simulink model "qpskUpdate"  (Simulink 9.2)
settings: Solver=FixedStepDiscrete  StartTime=0.0  StopTime=inf  RelTol=1e-3  AbsTol=1e-6
PreLoadFcn:
  | EbNo=3;maxNumErrs=100;maxNumBits=1e8;M=8;Tsym=.2;
model workspace: external: MATLAB Code (data not in the file)
libraries: commutil2 x2, commsink2 x2, commdigbbndpm3 x2, commchan3 x1, commrandsrc3 x1
Description:
  | Gray Coded 8-PSK
  | 
  | This model shows a communications link using Gray-coded 8-PSK modulation.
CloseFcn:
  | clear graySER grayBER graySigsOut EbNo maxNumErrs maxNumBits M Tsym
settings Model: RequirementInfo=9  Creator=The MathWorks, Inc.  LastModifiedBy=Milind  ExtModeTrigMode=oneshot  ExtModeArmWhenConnect=off  ExtModeAutoUpdateStatusClock=off
settings SolverCC: AutoScaleAbsTol=off
settings DataIOCC: LimitDataPoints=off  SignalLoggingSaveFormat=Dataset  SaveOutput=off  SaveTime=off  SignalLoggingName=graySigsOut
settings OptimizationCC: BlockReduction=off  BooleanDataType=off  ExpressionDepthLimit=2147483647  InitFltsAndDblsToZero=on  EfficientMapNaN2IntZero=off  BufferReusableBoundary=off
settings DebuggingCC: SaveWithParameterizedLinksMsg=none  CheckExecutionContextPreStartOutputMsg=on  CheckExecutionContextRuntimeOutputMsg=on  SignalResolutionControl=TryResolveAllWithWarning  MultiTaskDSMMsg=warning  MultiTaskCondExecSysMsg=none  SigSpecEnsureSampleTimeMsg=none  IntegerOverflowMsg=none  BusObjectLabelMismatch=none  LibraryContextMissingDiagnostic=none  IntegerSaturationMsg=none
settings HardwareCC: ProdHWDeviceType=Specified
settings ModelReferenceCC: UpdateModelReferenceTargets=IfOutOfDate
settings CodeAppCC: MangleLength=5
settings GRTTargetCC: TargetFcnLib=ansi_tfl_tmw.mat
settings ConfigComp: CovMetricSettings=d  CovSFcnEnable=off

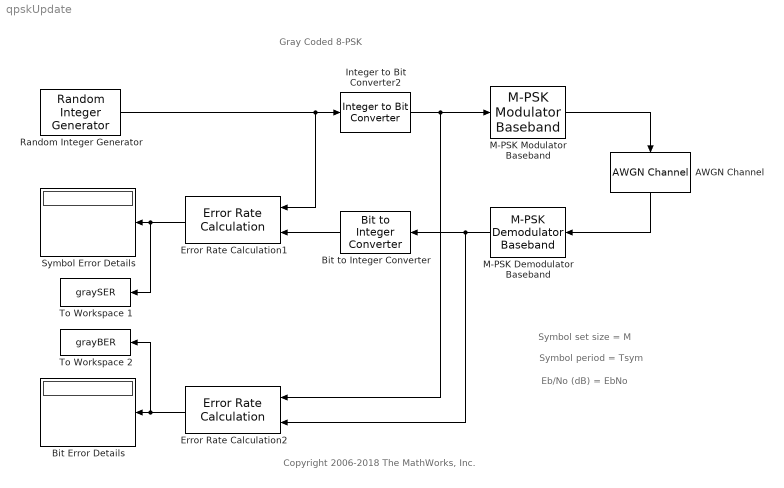
== system qpskUpdate ==
  note: Gray Coded 8-PSK
  note: Symbol set size = M
  note: Symbol period = Tsym
  note: Eb/No (dB) = EbNo
  note: Copyright 2006-2018 The MathWorks, Inc.
  AWGN Channel : commchan3/AWGN Channel  InputProcessing=Columns as channels (frame based)  seed=67  noiseMode="Signal to noise ratio  (Eb/No)"  EbNodB=EbNo  EsNodB=EbNo+10*log10(log2(M))  SNRdB=10  bitsPerSym=log2(4)  Ps=1  Tsym=0.001  variance=1
      settings: SourceProductName=Communications Toolbox
  Bit Error Details : Display
  Bit to Integer Converter : commutil2/Bit to Integer Converter  nbits=log2(4)  bitOrder=MSB first  signedOutputValues=Unsigned  outDtype=Smallest integer  outDtypeSigned=Inherit via internal rule
      settings: SourceProductName=Communications Toolbox
  Error Rate Calculation1 : commsink2/Error Rate Calculation  N=0  st_delay=0  cp_mode=Entire frame  subframe=[]  PMode=Port  WsName=SymErrorVec  RsMode2=off  stop=off  numErr=100  maxBits=1e6
      settings: SourceProductName=Communications Toolbox
  Error Rate Calculation2 : commsink2/Error Rate Calculation  N=0  st_delay=0  cp_mode=Entire frame  subframe=[]  PMode=Port  WsName=BitErrorVec  RsMode2=off  stop=on  numErr=maxNumErrs  maxBits=maxNumBits
      settings: SourceProductName=Communications Toolbox
  Integer to Bit Converter2 : commutil2/Integer to Bit Converter  nbits=log2(4)  signedInputValues=Unsigned  bitOrder=MSB first  outDtype=Smallest unsigned integer
      settings: SourceProductName=Communications Toolbox
  M-PSK Demodulator Baseband : commdigbbndpm3/M-PSK Demodulator Baseband  M=4  OutType=Bit  DecType=Hard decision  VarSource=Dialog  Variance=1  Dec=Gray  Mapping=[0:7]  Ph=0  outDtype1=Smallest unsigned integer  outDtype2=double  derotateFactorWordLen=16  derotateFactorDataTypeStr=Inherit: Same word length as input  derotateFactorLastDataTypeStr=Inherit: Same word length as input
      settings: SourceProductName=Communications Toolbox
  M-PSK Modulator Baseband : commdigbbndpm3/M-PSK Modulator Baseband  M=4  InType=Bit  Enc=Gray  Mapping=0  Ph=0  outDtype=double  outWordLen=16  outUDDataType=sfix(16)  outFracLenMode=Best precision  outFracLen=15  outDataTypeStr=double  outLastDataTypeStr=double
      settings: SourceProductName=Communications Toolbox
  Random Integer Generator : commrandsrc3/Random Integer Generator  SetSize=4  SeedSource=Parameter  Seed=529558  SampleTime=0.001  SamplesPerFrame=100  OutputDataType=uint8  SimulateUsing=Interpreted execution
      settings: SourceProductName=Communications Toolbox
  Symbol Error Details : Display
  To Workspace 1 : ToWorkspace  VariableName=graySER  SampleTime=-1
      settings: MaxDataPoints=1
  To Workspace 2 : ToWorkspace  VariableName=grayBER  SampleTime=-1
      settings: MaxDataPoints=1
  wires:
  Error Rate Calculation2/1 -> Bit Error Details/1, To Workspace 2/1
  Error Rate Calculation1/1 -> Symbol Error Details/1, To Workspace 1/1
  M-PSK Demodulator Baseband/1 -> Bit to Integer Converter/1, Error Rate Calculation2/2
  Random Integer Generator/1 -> Integer to Bit Converter2/1, Error Rate Calculation1/1
  AWGN Channel/1 -> M-PSK Demodulator Baseband/1
  M-PSK Modulator Baseband/1 -> AWGN Channel/1
  Integer to Bit Converter2/1 -> Error Rate Calculation2/1, M-PSK Modulator Baseband/1
  Bit to Integer Converter/1 -> Error Rate Calculation1/2
